simulink model "AM_07_model_pretvornik_FOC"  (R2016a)
settings: Solver=ode23  StartTime=0.0  StopTime=1  FixedStep=25e-9  MaxStep=1/(20*Fstikalna)  RelTol=1e-2
InitFcn:
  | parametriAM
values from neighbouring files (symbols this model uses):
  Imrn = 7.4    [parametriAM.m]
  In = 12.7    [parametriAM.m]
  Ismax = In*sqrt(2)    [parametriAM.m]
  J = 0.019    [parametriAM.m]    (also in podatki.m = 0.01)
  Ki_tok = 5.0    (= 5)    [parametriAM.m]
  Ki_wr = 1000    [parametriAM.m]
  Kp_tok = 0.05    [parametriAM.m]
  Kp_wr = 50    [parametriAM.m]
  Lm = 0.0493    [parametriAM.m]    (also in podatki.m = 0.2342)
  Lr = 0.05315    [parametriAM.m]    (also in podatki.m = 0.2449)
  Ls = 0.05315    [parametriAM.m]    (also in podatki.m = 0.2449)
  Lst = sigma*Ls    (= 0.00742111947319)    [parametriAM.m]
  pp = 3    [parametriAM.m]    (also in podatki.m = 2)
  sigma = 1 - 1/((1+sigmaR)*(1+sigmaS))    (= 0.13962595434)    [parametriAM.m]
  Tr = Lr/Rr    (= 0.0771407837446)    [parametriAM.m]
  Tstikalna = 1/Fstikalna    (= 0.0001)    [parametriAM.m]
  Udc = Un*sqrt(2/3*2)    [parametriAM.m]
  Un = 216    [parametriAM.m]
  wb_upper_limit_field_weaking = sqrt((Ls^2+Lst^2)/(2*Lst^2*Ls^2))*Un/Ismax    [parametriAM.m]
  wn = Udc/sqrt(Ls^2*(Imrn)^2+Lst^2*(Ismax^2-(Imrn)^2))    [maximalnaelipsa.m]    (also in parametriAM.m = Udc/sqrt(Ls^2*(Imrn)^2+Lst^2*(Ismax^2-(Imrn)^2))/pp/sqrt(2))
undefined symbols (not defined in the file or in its folder): DiscIntNeverNeededParam
undefined symbols (not defined in the file): Rr, Rs
libraries: simulink x23, simulink_extras x3
(part 1 of 2)
settings Model: Creator=Mitja  LastModifiedBy=Mitja1
settings DataIOCC: LimitDataPoints=on  SaveFormat=Array  SignalLoggingSaveFormat=ModelDataLogs
settings OptimizationCC: ExpressionDepthLimit=2147483647  InitFltsAndDblsToZero=on
settings DebuggingCC: SaveWithParameterizedLinksMsg=none  UnderspecifiedInitializationDetection=Classic  MergeDetectMultiDrivingBlocksExec=none  SignalResolutionControl=TryResolveAllWithWarning  SolverPrmCheckMsg=warning  FcnCallInpInsideContextMsg=UseLocalSettings  StateNameClashWarn=warning  StrictBusMsg=Warning
settings HardwareCC: ProdBitPerPointer=32  ProdLargestAtomicFloat=None  ProdIntDivRoundTo=Undefined  ProdEndianess=Unspecified  ProdWordSize=32  ProdHWDeviceType=32-bit Generic
settings ModelReferenceCC: PropagateSignalLabelsOutOfModel=off
settings GRTTargetCC: TargetFcnLib=ansi_tfl_tmw.mat  CombineOutputUpdateFcns=off  GRTInterface=on
settings ConfigComp: CovModelRefEnable=Off

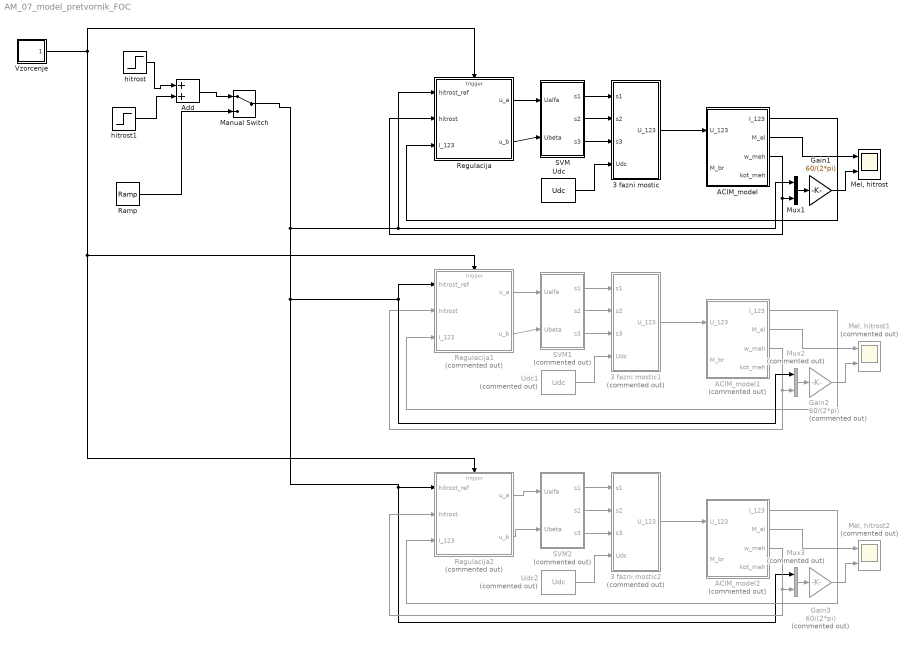
== system AM_07_model_pretvornik_FOC ==
  3 fazni mostic : Subsystem
  3 fazni mostic1 : Subsystem  Commented=on
  3 fazni mostic2 : Subsystem  Commented=on
  ACIM_model : Subsystem  mask{R_s=Rs, R_r=Rr, L_s=Ls, L_r=Lr, L_m=Lm, sigma=sigma, pp=pp, J=J, Ktrenja=0, Kupora=0}
      mask prompts: R_s "Statorska upornost"; R_r "Rotorska upornost"; L_s "Statorska induktivnost"; L_r "Rotorska induktivnost"; L_m "Medsebojna induktivnost"; sigma "Fakstor stresanja"; pp "Število polovih parov"; J "Mehanska vztrajnost"; Ktrenja "Koeficient trenja"; Kupora "Koeficient upora"
  ACIM_model1 : Subsystem  Commented=on  mask{R_s=Rs, R_r=Rr, L_s=Ls, L_r=Lr, L_m=Lm, sigma=sigma, pp=pp, J=J, Ktrenja=0, Kupora=0}
      mask prompts: R_s "Statorska upornost"; R_r "Rotorska upornost"; L_s "Statorska induktivnost"; L_r "Rotorska induktivnost"; L_m "Medsebojna induktivnost"; sigma "Fakstor stresanja"; pp "Število polovih parov"; J "Mehanska vztrajnost"; Ktrenja "Koeficient trenja"; Kupora "Koeficient upora"
  ACIM_model2 : Subsystem  Commented=on  mask{R_s=Rs, R_r=Rr, L_s=Ls, L_r=Lr, L_m=Lm, sigma=sigma, pp=pp, J=J, Ktrenja=0, Kupora=0}
      mask prompts: R_s "Statorska upornost"; R_r "Rotorska upornost"; L_s "Statorska induktivnost"; L_r "Rotorska induktivnost"; L_m "Medsebojna induktivnost"; sigma "Fakstor stresanja"; pp "Število polovih parov"; J "Mehanska vztrajnost"; Ktrenja "Koeficient trenja"; Kupora "Koeficient upora"
  Add : Sum
  Gain1 : Gain  Gain=60/(2*pi)
  Gain2 : Gain  Commented=on  Gain=60/(2*pi)
  Gain3 : Gain  Commented=on  Gain=60/(2*pi)
  Manual Switch : ManualSwitch
  "Mel, hitrost" : Scope  NumInputPorts=2
  "Mel, hitrost1" : Scope  Commented=on  NumInputPorts=2
  "Mel, hitrost2" : Scope  Commented=on  NumInputPorts=2
  Mux1 : Mux  Inputs=2
  Mux2 : Mux  Commented=on  Inputs=2
  Mux3 : Mux  Commented=on  Inputs=2
  Ramp : simulink/Sources/Ramp  slope=1  start=0  X0=0
  Regulacija : Subsystem  TreatAsAtomicUnit=on
  Regulacija1 : Subsystem  Commented=on  TreatAsAtomicUnit=on
  Regulacija2 : Subsystem  Commented=on  TreatAsAtomicUnit=on
  SVM : Subsystem
  SVM1 : Subsystem  Commented=on
  SVM2 : Subsystem  Commented=on
  Udc : Constant  Value=Udc
  Udc1 : Constant  Commented=on  Value=Udc
  Udc2 : Constant  Commented=on  Value=Udc
  Vzorcenje : Subsystem
  hitrost : Step  Time=0.1  After=(2000)*2*pi/60  SampleTime=0
  hitrost1 : Step  Time=0.3  After=2000*2*pi/60  SampleTime=0
  wires:
  Udc/1 -> 3 fazni mostic/4(Udc)
  SVM/1(s1) -> 3 fazni mostic/1(s1)
  SVM/2(s2) -> 3 fazni mostic/2(s2)
  SVM/3(s3) -> 3 fazni mostic/3(s3)
  Regulacija/1(u_a) -> SVM/1(Ualfa)
  Regulacija/2(u_b) -> SVM/2(Ubeta)
  3 fazni mostic/1(U_123) -> ACIM_model/1(U_123)
  hitrost/1 -> Add/1
  ACIM_model/1(I_123) -> Regulacija/3(I_123)
  ACIM_model/2(M_el) -> "Mel, hitrost"/1
  ACIM_model/3(w_meh) -> Mux1/2, Regulacija/2(hitrost)
  Gain1/1 -> "Mel, hitrost"/2
  Mux1/1 -> Gain1/1
  Udc1/1 -> 3 fazni mostic1/4(Udc)
  SVM1/1(s1) -> 3 fazni mostic1/1(s1)
  SVM1/2(s2) -> 3 fazni mostic1/2(s2)
  SVM1/3(s3) -> 3 fazni mostic1/3(s3)
  Regulacija1/1(u_a) -> SVM1/1(Ualfa)
  Regulacija1/2(u_b) -> SVM1/2(Ubeta)
  3 fazni mostic1/1(U_123) -> ACIM_model1/1(U_123)
  ACIM_model1/1(I_123) -> Regulacija1/3(I_123)
  ACIM_model1/2(M_el) -> "Mel, hitrost1"/1
  ACIM_model1/3(w_meh) -> Regulacija1/2(hitrost), Mux2/2
  Gain2/1 -> "Mel, hitrost1"/2
  Mux2/1 -> Gain2/1
  Udc2/1 -> 3 fazni mostic2/4(Udc)
  SVM2/1(s1) -> 3 fazni mostic2/1(s1)
  SVM2/2(s2) -> 3 fazni mostic2/2(s2)
  SVM2/3(s3) -> 3 fazni mostic2/3(s3)
  Regulacija2/1(u_a) -> SVM2/1(Ualfa)
  Regulacija2/2(u_b) -> SVM2/2(Ubeta)
  3 fazni mostic2/1(U_123) -> ACIM_model2/1(U_123)
  Manual Switch/1 -> Mux3/1, Regulacija2/1(hitrost_ref), Mux2/1, Regulacija1/1(hitrost_ref), Regulacija/1(hitrost_ref), Mux1/1
  ACIM_model2/1(I_123) -> Regulacija2/3(I_123)
  ACIM_model2/2(M_el) -> "Mel, hitrost2"/1
  ACIM_model2/3(w_meh) -> Mux3/2, Regulacija2/2(hitrost)
  Vzorcenje/1(trigger) -> Regulacija/Trigger, Regulacija2/Trigger, Regulacija1/Trigger
  Gain3/1 -> "Mel, hitrost2"/2
  Mux3/1 -> Gain3/1
  Ramp/1 -> Manual Switch/2
  Add/1 -> Manual Switch/1
  hitrost1/1 -> Add/2

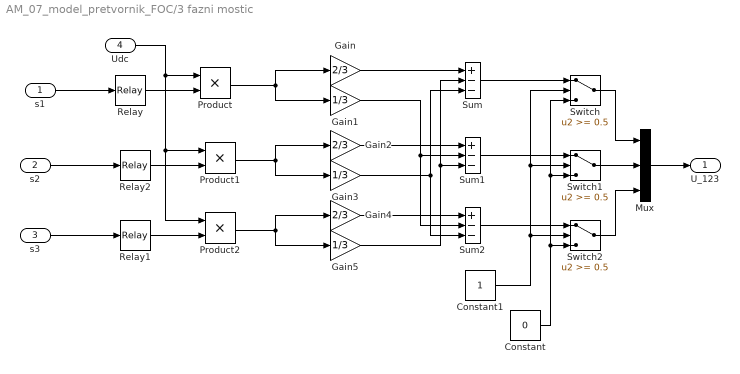
== system AM_07_model_pretvornik_FOC/3 fazni mostic ==
  s1 : Inport
  s2 : Inport  Port=2
  s3 : Inport  Port=3
  Udc : Inport  Port=4
  Constant : Constant  Value=0
  Constant1 : Constant
  Gain : Gain  Gain=2/3
  Gain1 : Gain  Gain=1/3
  Gain2 : Gain  Gain=2/3
  Gain3 : Gain  Gain=1/3
  Gain4 : Gain  Gain=2/3
  Gain5 : Gain  Gain=1/3
  Mux : Mux  Inputs=3
  Product : Product  RndMeth=Zero
  Product1 : Product  RndMeth=Zero
  Product2 : Product  RndMeth=Zero
  Relay : Relay  OnSwitchValue=0.5  OffSwitchValue=0.5  OnOutputValue=0.5  OffOutputValue=-0.5
  Relay1 : Relay  OnSwitchValue=0.5  OffSwitchValue=0.5  OnOutputValue=0.5  OffOutputValue=-0.5
  Relay2 : Relay  OnSwitchValue=0.5  OffSwitchValue=0.5  OnOutputValue=0.5  OffOutputValue=-0.5
  Sum : Sum  Inputs=+--
  Sum1 : Sum  Inputs=+--
  Sum2 : Sum  Inputs=+--
  Switch : Switch  Threshold=0.5
  Switch1 : Switch  Threshold=0.5
  Switch2 : Switch  Threshold=0.5
  U_123 : Outport
  wires:
  Constant/1 -> Switch2/3, Switch1/3, Switch/3
  Constant1/1 -> Switch2/2, Switch1/2, Switch/2
  Udc/1 -> Product/1, Product1/1, Product2/1
  Sum/1 -> Switch/1
  Sum1/1 -> Switch1/1
  Sum2/1 -> Switch2/1
  Product/1 -> Gain/1, Gain1/1
  Product1/1 -> Gain2/1, Gain3/1
  Product2/1 -> Gain4/1, Gain5/1
  Gain/1 -> Sum/1
  Gain2/1 -> Sum1/1
  Gain4/1 -> Sum2/1
  Gain1/1 -> Sum2/2, Sum1/2
  Gain3/1 -> Sum2/3, Sum/3
  Gain5/1 -> Sum/2, Sum1/3
  Relay/1 -> Product/2
  Relay2/1 -> Product1/2
  Relay1/1 -> Product2/2
  s3/1 -> Relay1/1
  s1/1 -> Relay/1
  s2/1 -> Relay2/1
  Switch1/1 -> Mux/2
  Switch/1 -> Mux/1
  Switch2/1 -> Mux/3
  Mux/1 -> U_123/1

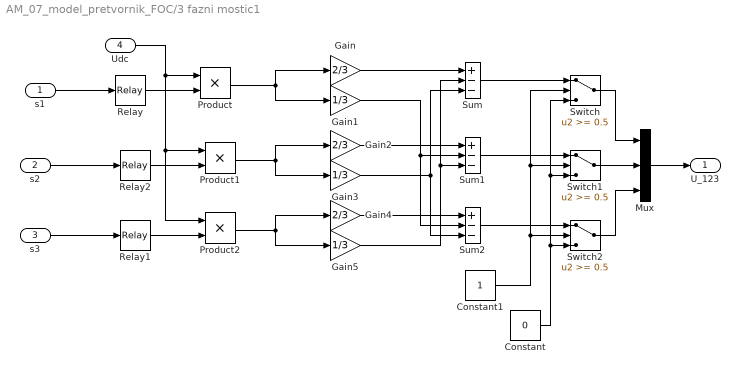
== system AM_07_model_pretvornik_FOC/3 fazni mostic1 ==
  s1 : Inport
  s2 : Inport  Port=2
  s3 : Inport  Port=3
  Udc : Inport  Port=4
  Constant : Constant  Value=0
  Constant1 : Constant
  Gain : Gain  Gain=2/3
  Gain1 : Gain  Gain=1/3
  Gain2 : Gain  Gain=2/3
  Gain3 : Gain  Gain=1/3
  Gain4 : Gain  Gain=2/3
  Gain5 : Gain  Gain=1/3
  Mux : Mux  Inputs=3
  Product : Product  RndMeth=Zero
  Product1 : Product  RndMeth=Zero
  Product2 : Product  RndMeth=Zero
  Relay : Relay  OnSwitchValue=0.5  OffSwitchValue=0.5  OnOutputValue=0.5  OffOutputValue=-0.5
  Relay1 : Relay  OnSwitchValue=0.5  OffSwitchValue=0.5  OnOutputValue=0.5  OffOutputValue=-0.5
  Relay2 : Relay  OnSwitchValue=0.5  OffSwitchValue=0.5  OnOutputValue=0.5  OffOutputValue=-0.5
  Sum : Sum  Inputs=+--
  Sum1 : Sum  Inputs=+--
  Sum2 : Sum  Inputs=+--
  Switch : Switch  Threshold=0.5
  Switch1 : Switch  Threshold=0.5
  Switch2 : Switch  Threshold=0.5
  U_123 : Outport
  wires:
  Mux/1 -> U_123/1
  Switch2/1 -> Mux/3
  Switch/1 -> Mux/1
  Switch1/1 -> Mux/2
  s2/1 -> Relay2/1
  s1/1 -> Relay/1
  s3/1 -> Relay1/1
  Relay1/1 -> Product2/2
  Relay2/1 -> Product1/2
  Relay/1 -> Product/2
  Gain5/1 -> Sum1/3, Sum/2
  Gain3/1 -> Sum/3, Sum2/3
  Gain1/1 -> Sum1/2, Sum2/2
  Gain4/1 -> Sum2/1
  Gain2/1 -> Sum1/1
  Gain/1 -> Sum/1
  Product2/1 -> Gain5/1, Gain4/1
  Product1/1 -> Gain3/1, Gain2/1
  Product/1 -> Gain1/1, Gain/1
  Sum2/1 -> Switch2/1
  Sum1/1 -> Switch1/1
  Sum/1 -> Switch/1
  Udc/1 -> Product2/1, Product1/1, Product/1
  Constant1/1 -> Switch/2, Switch1/2, Switch2/2
  Constant/1 -> Switch/3, Switch1/3, Switch2/3

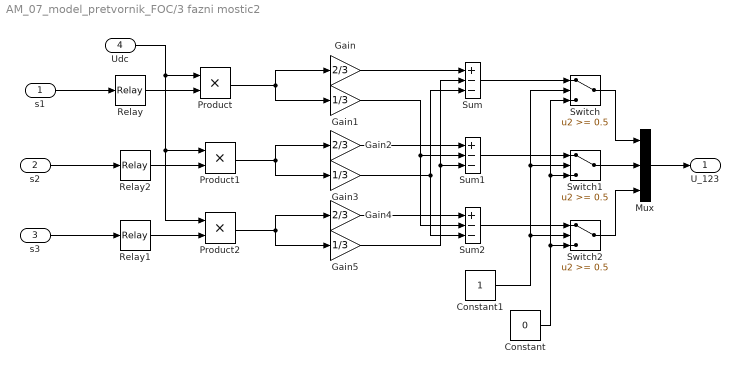
== system AM_07_model_pretvornik_FOC/3 fazni mostic2 ==
  s1 : Inport
  s2 : Inport  Port=2
  s3 : Inport  Port=3
  Udc : Inport  Port=4
  Constant : Constant  Value=0
  Constant1 : Constant
  Gain : Gain  Gain=2/3
  Gain1 : Gain  Gain=1/3
  Gain2 : Gain  Gain=2/3
  Gain3 : Gain  Gain=1/3
  Gain4 : Gain  Gain=2/3
  Gain5 : Gain  Gain=1/3
  Mux : Mux  Inputs=3
  Product : Product  RndMeth=Zero
  Product1 : Product  RndMeth=Zero
  Product2 : Product  RndMeth=Zero
  Relay : Relay  OnSwitchValue=0.5  OffSwitchValue=0.5  OnOutputValue=0.5  OffOutputValue=-0.5
  Relay1 : Relay  OnSwitchValue=0.5  OffSwitchValue=0.5  OnOutputValue=0.5  OffOutputValue=-0.5
  Relay2 : Relay  OnSwitchValue=0.5  OffSwitchValue=0.5  OnOutputValue=0.5  OffOutputValue=-0.5
  Sum : Sum  Inputs=+--
  Sum1 : Sum  Inputs=+--
  Sum2 : Sum  Inputs=+--
  Switch : Switch  Threshold=0.5
  Switch1 : Switch  Threshold=0.5
  Switch2 : Switch  Threshold=0.5
  U_123 : Outport
  wires:
  Constant/1 -> Switch2/3, Switch1/3, Switch/3
  Constant1/1 -> Switch2/2, Switch1/2, Switch/2
  Udc/1 -> Product/1, Product1/1, Product2/1
  Sum/1 -> Switch/1
  Sum1/1 -> Switch1/1
  Sum2/1 -> Switch2/1
  Product/1 -> Gain/1, Gain1/1
  Product1/1 -> Gain2/1, Gain3/1
  Product2/1 -> Gain4/1, Gain5/1
  Gain/1 -> Sum/1
  Gain2/1 -> Sum1/1
  Gain4/1 -> Sum2/1
  Gain1/1 -> Sum2/2, Sum1/2
  Gain3/1 -> Sum2/3, Sum/3
  Gain5/1 -> Sum/2, Sum1/3
  Relay/1 -> Product/2
  Relay2/1 -> Product1/2
  Relay1/1 -> Product2/2
  s3/1 -> Relay1/1
  s1/1 -> Relay/1
  s2/1 -> Relay2/1
  Switch1/1 -> Mux/2
  Switch/1 -> Mux/1
  Switch2/1 -> Mux/3
  Mux/1 -> U_123/1

== system AM_07_model_pretvornik_FOC/ACIM_model ==
  U_123 : Inport
  M_br : Inport  Port=2
  Elektricni del1 : Subsystem  mask{Rs=R_s, Rr=R_r, Ls=L_s, Lr=L_r, Lm=L_m, sigma=sigma, pp=pp}
      mask prompts: Rs "Statorska upornost"; Rr "Rotorska upornost"; Ls "Statorska induktivnost"; Lr "Statorska induktivnost"; Lm "Medsebojna induktivnost"; sigma "Faktor stresanja sigma"; pp "Število polovih parov"
  Mehanika : Subsystem  mask{J=J, Ktrenja=Ktrenja, Kupora=Kupora}
      mask prompts: J "Rotacijska vztrajnost"; Ktrenja "Koeficient trenja"; Kupora "Koeficient zracnega upora"
  I_123 : Outport
  M_el : Outport  Port=2
  w_meh : Outport  Port=3
  kot_meh : Outport  Port=4
  wires:
  Mehanika/1(w_meh) -> Elektricni del1/2(w_meh), w_meh/1
  Mehanika/2(kot_meh) -> kot_meh/1
  Elektricni del1/2(I_123) -> I_123/1
  U_123/1 -> Elektricni del1/1(U_123)
  M_br/1 -> Mehanika/2(M_br)
  Elektricni del1/1(Mel) -> M_el/1, Mehanika/1(M_el)

== system AM_07_model_pretvornik_FOC/ACIM_model1 ==
  U_123 : Inport
  M_br : Inport  Port=2
  Elektricni del1 : Subsystem  mask{Rs=R_s, Rr=R_r, Ls=L_s, Lr=L_r, Lm=L_m, sigma=sigma, pp=pp}
      mask prompts: Rs "Statorska upornost"; Rr "Rotorska upornost"; Ls "Statorska induktivnost"; Lr "Statorska induktivnost"; Lm "Medsebojna induktivnost"; sigma "Faktor stresanja sigma"; pp "Število polovih parov"
  Mehanika : Subsystem  mask{J=J, Ktrenja=Ktrenja, Kupora=Kupora}
      mask prompts: J "Rotacijska vztrajnost"; Ktrenja "Koeficient trenja"; Kupora "Koeficient zracnega upora"
  I_123 : Outport
  M_el : Outport  Port=2
  w_meh : Outport  Port=3
  kot_meh : Outport  Port=4
  wires:
  Elektricni del1/1(Mel) -> Mehanika/1(M_el), M_el/1
  M_br/1 -> Mehanika/2(M_br)
  U_123/1 -> Elektricni del1/1(U_123)
  Elektricni del1/2(I_123) -> I_123/1
  Mehanika/2(kot_meh) -> kot_meh/1
  Mehanika/1(w_meh) -> w_meh/1, Elektricni del1/2(w_meh)

== system AM_07_model_pretvornik_FOC/ACIM_model2 ==
  U_123 : Inport
  M_br : Inport  Port=2
  Elektricni del1 : Subsystem  mask{Rs=R_s, Rr=R_r, Ls=L_s, Lr=L_r, Lm=L_m, sigma=sigma, pp=pp}
      mask prompts: Rs "Statorska upornost"; Rr "Rotorska upornost"; Ls "Statorska induktivnost"; Lr "Statorska induktivnost"; Lm "Medsebojna induktivnost"; sigma "Faktor stresanja sigma"; pp "Število polovih parov"
  Mehanika : Subsystem  mask{J=J, Ktrenja=Ktrenja, Kupora=Kupora}
      mask prompts: J "Rotacijska vztrajnost"; Ktrenja "Koeficient trenja"; Kupora "Koeficient zracnega upora"
  I_123 : Outport
  M_el : Outport  Port=2
  w_meh : Outport  Port=3
  kot_meh : Outport  Port=4
  wires:
  Mehanika/1(w_meh) -> Elektricni del1/2(w_meh), w_meh/1
  Mehanika/2(kot_meh) -> kot_meh/1
  Elektricni del1/2(I_123) -> I_123/1
  U_123/1 -> Elektricni del1/1(U_123)
  M_br/1 -> Mehanika/2(M_br)
  Elektricni del1/1(Mel) -> M_el/1, Mehanika/1(M_el)

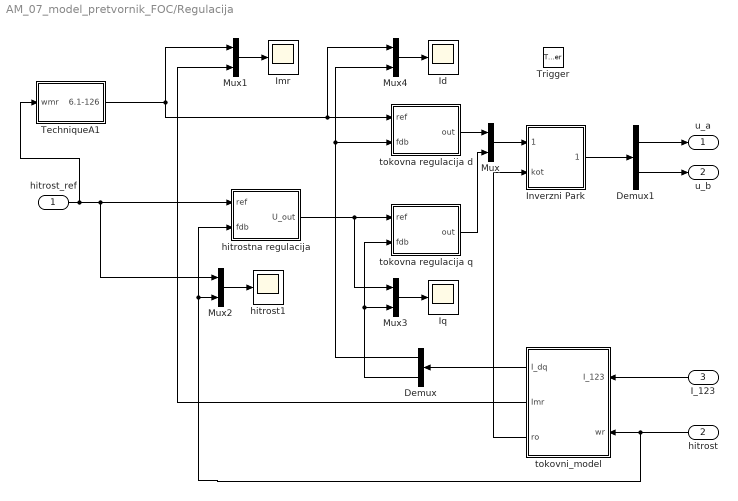
== system AM_07_model_pretvornik_FOC/Regulacija ==
  hitrost_ref : Inport
  hitrost : Inport  Port=2
  I_123 : Inport  Port=3
  Trigger : TriggerPort  TriggerType=falling  VariantControl=Variant
  Demux : Demux  Outputs=2
  Demux1 : Demux  Outputs=2
  Id : Scope
  Imr : Scope
  Inverzni Park : Subsystem
  Iq : Scope
  Mux{,1..4} (5 alike) : Mux  Inputs=2
  TechniqueA1 : Subsystem
  hitrost1 : Scope
  hitrostna regulacija : Subsystem
  tokovna regulacija d : Subsystem
  tokovna regulacija q : Subsystem
  tokovni_model : Subsystem
  u_a : Outport
  u_b : Outport  Port=2
  wires:
  I_123/1 -> tokovni_model/1(I_123)
  hitrost/1 -> Mux2/2, hitrostna regulacija/2(fdb), tokovni_model/2(wr)
  tokovni_model/3(ro) -> Inverzni Park/2(kot)
  hitrost_ref/1 -> TechniqueA1/1(wmr), hitrostna regulacija/1(ref), Mux2/1
  Mux/1 -> Inverzni Park/1(U_dq)
  TechniqueA1/1(6.1-126) -> tokovna regulacija d/1(ref), Mux4/1, Mux1/1
  tokovna regulacija d/1(out) -> Mux/1
  tokovna regulacija q/1(out) -> Mux/2
  Demux/1 -> tokovna regulacija d/2(fdb), Mux4/2
  Demux/2 -> Mux3/2, tokovna regulacija q/2(fdb)
  Inverzni Park/1(U_ab) -> Demux1/1
  Demux1/1 -> u_a/1
  Demux1/2 -> u_b/1
  Mux1/1 -> Imr/1
  Mux2/1 -> hitrost1/1
  Mux3/1 -> Iq/1
  Mux4/1 -> Id/1
  tokovni_model/2(Imr) -> Mux1/2
  tokovni_model/1(I_dq) -> Demux/1
  hitrostna regulacija/1(U_out) -> tokovna regulacija q/1(ref), Mux3/1

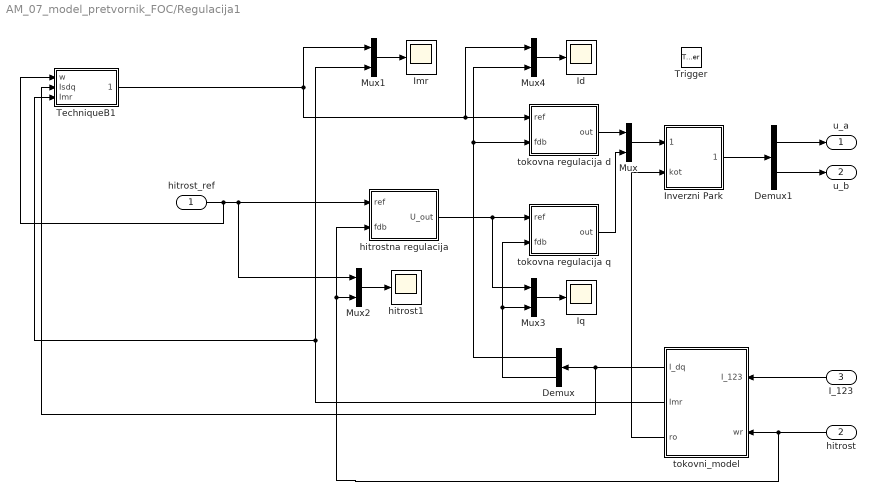
== system AM_07_model_pretvornik_FOC/Regulacija1 ==
  hitrost_ref : Inport
  hitrost : Inport  Port=2
  I_123 : Inport  Port=3
  Trigger : TriggerPort  TriggerType=falling  VariantControl=Variant
  Demux : Demux  Outputs=2
  Demux1 : Demux  Outputs=2
  Id : Scope
  Imr : Scope
  Inverzni Park : Subsystem
  Iq : Scope
  Mux{,1..4} (5 alike) : Mux  Inputs=2
  TechniqueB1 : Subsystem
  hitrost1 : Scope
  hitrostna regulacija : Subsystem
  tokovna regulacija d : Subsystem
  tokovna regulacija q : Subsystem
  tokovni_model : Subsystem
  u_a : Outport
  u_b : Outport  Port=2
  wires:
  hitrostna regulacija/1(U_out) -> Mux3/1, tokovna regulacija q/1(ref)
  tokovni_model/1(I_dq) -> TechniqueB1/2(Isdq), Demux/1
  tokovni_model/2(Imr) -> TechniqueB1/3(Imr), Mux1/2
  Mux4/1 -> Id/1
  Mux3/1 -> Iq/1
  Mux2/1 -> hitrost1/1
  Mux1/1 -> Imr/1
  Demux1/2 -> u_b/1
  Demux1/1 -> u_a/1
  Inverzni Park/1(U_ab) -> Demux1/1
  Demux/2 -> tokovna regulacija q/2(fdb), Mux3/2
  Demux/1 -> Mux4/2, tokovna regulacija d/2(fdb)
  tokovna regulacija q/1(out) -> Mux/2
  tokovna regulacija d/1(out) -> Mux/1
  TechniqueB1/1(6.1-135) -> Mux4/1, tokovna regulacija d/1(ref), Mux1/1
  Mux/1 -> Inverzni Park/1(U_dq)
  hitrost_ref/1 -> TechniqueB1/1(w), Mux2/1, hitrostna regulacija/1(ref)
  tokovni_model/3(ro) -> Inverzni Park/2(kot)
  hitrost/1 -> tokovni_model/2(wr), hitrostna regulacija/2(fdb), Mux2/2
  I_123/1 -> tokovni_model/1(I_123)

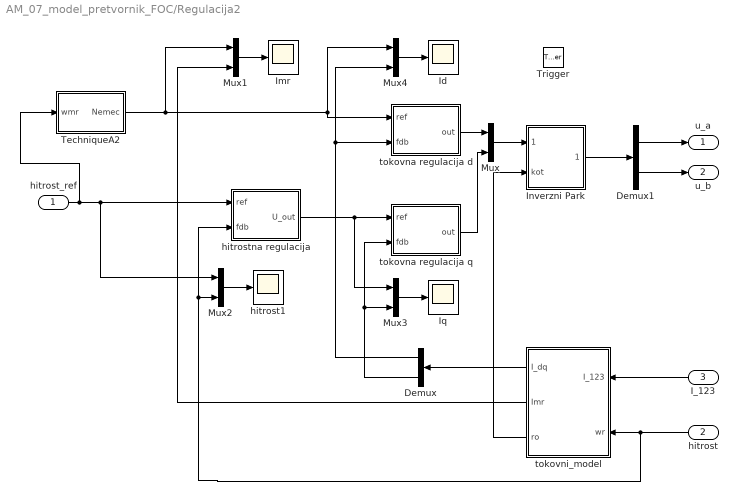
== system AM_07_model_pretvornik_FOC/Regulacija2 ==
  hitrost_ref : Inport
  hitrost : Inport  Port=2
  I_123 : Inport  Port=3
  Trigger : TriggerPort  TriggerType=falling  VariantControl=Variant
  Demux : Demux  Outputs=2
  Demux1 : Demux  Outputs=2
  Id : Scope
  Imr : Scope
  Inverzni Park : Subsystem
  Iq : Scope
  Mux{,1..4} (5 alike) : Mux  Inputs=2
  TechniqueA2 : Subsystem
  hitrost1 : Scope
  hitrostna regulacija : Subsystem
  tokovna regulacija d : Subsystem
  tokovna regulacija q : Subsystem
  tokovni_model : Subsystem
  u_a : Outport
  u_b : Outport  Port=2
  wires:
  I_123/1 -> tokovni_model/1(I_123)
  hitrost/1 -> Mux2/2, hitrostna regulacija/2(fdb), tokovni_model/2(wr)
  tokovni_model/3(ro) -> Inverzni Park/2(kot)
  hitrost_ref/1 -> TechniqueA2/1(wmr), hitrostna regulacija/1(ref), Mux2/1
  Mux/1 -> Inverzni Park/1(U_dq)
  TechniqueA2/1(Nemec) -> tokovna regulacija d/1(ref), Mux4/1, Mux1/1
  tokovna regulacija d/1(out) -> Mux/1
  tokovna regulacija q/1(out) -> Mux/2
  Demux/1 -> tokovna regulacija d/2(fdb), Mux4/2
  Demux/2 -> Mux3/2, tokovna regulacija q/2(fdb)
  Inverzni Park/1(U_ab) -> Demux1/1
  Demux1/1 -> u_a/1
  Demux1/2 -> u_b/1
  Mux1/1 -> Imr/1
  Mux2/1 -> hitrost1/1
  Mux3/1 -> Iq/1
  Mux4/1 -> Id/1
  tokovni_model/2(Imr) -> Mux1/2
  tokovni_model/1(I_dq) -> Demux/1
  hitrostna regulacija/1(U_out) -> tokovna regulacija q/1(ref), Mux3/1

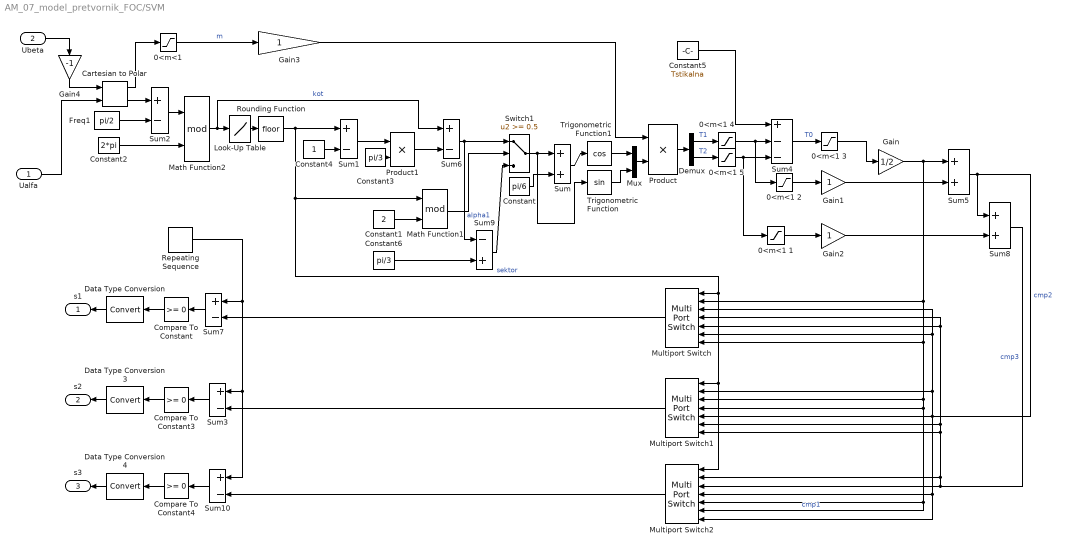
== system AM_07_model_pretvornik_FOC/SVM ==
  Ualfa : Inport
  Ubeta : Inport  Port=2
  "0<m<1 " : Saturate  UpperLimit=0.99  LowerLimit=0
  0<m<1 {1..5} (5 alike) : Saturate  UpperLimit=1  LowerLimit=0
  Cartesian to Polar : simulink_extras/Transformations/Cartesian to Polar
  Compare To Constant : simulink/Logic and Bit Operations/Compare To Constant  relop=>=  const=0  OutDataTypeStr=uint8  ZeroCross=off
  Compare To Constant3 : simulink/Logic and Bit Operations/Compare To Constant  relop=>=  const=0  OutDataTypeStr=uint8  ZeroCross=off
  Compare To Constant4 : simulink/Logic and Bit Operations/Compare To Constant  relop=>=  const=0  OutDataTypeStr=uint8  ZeroCross=off
  Constant : Constant  Value=pi/6
  Constant1 : Constant  Value=2
  Constant2 : Constant  Value=2*pi
  Constant3 : Constant  Value=pi/3
  Constant4 : Constant
  Constant5 : Constant  Value=Tstikalna
  Constant6 : Constant  Value=pi/3
  Data Type Conversion : DataTypeConversion
  Data Type Conversion3 : DataTypeConversion
  Data Type Conversion4 : DataTypeConversion
  Demux : Demux  Outputs=2
  Freq1 : Constant  Value=pi/2
  Gain : Gain  Gain=1/2
  Gain1 : Gain
  Gain2 : Gain
  Gain3 : Gain
  Gain4 : Gain  Gain=-1
  Look-Up Table : Lookup  InputValues=[0:pi/3:5*pi/3]  Table=[1:6]  SaturateOnIntegerOverflow=on
  Math Function1 : Math  Operator=mod  SaturateOnIntegerOverflow=on
  Math Function2 : Math  Operator=mod  SaturateOnIntegerOverflow=on
  Multiport Switch : MultiPortSwitch  Inputs=6  DiagnosticForDefault=Warning
  Multiport Switch1 : MultiPortSwitch  Inputs=6  DiagnosticForDefault=Warning
  Multiport Switch2 : MultiPortSwitch  Inputs=6  DiagnosticForDefault=Warning
  Mux : Mux  Inputs=2
  Product : Product  SaturateOnIntegerOverflow=on  OutDataTypeStr=Inherit: Same as first input
  Product1 : Product  SaturateOnIntegerOverflow=on  OutDataTypeStr=Inherit: Same as first input
  Repeating Sequence : simulink/Sources/Repeating Sequence  rep_seq_t=[0 Tstikalna/2 Tstikalna]  rep_seq_y=[0 1 0]
  Rounding Function : Rounding
  Sum : Sum  SaturateOnIntegerOverflow=on
  Sum1 : Sum  Inputs=+-  SaturateOnIntegerOverflow=on
  Sum10 : Sum  Inputs=+-
  Sum2 : Sum  Inputs=+-  SaturateOnIntegerOverflow=on  InputSameDT=on  OutDataTypeStr=Inherit: Same as first input
  Sum3 : Sum  Inputs=+-
  Sum4 : Sum  Inputs=+--  SaturateOnIntegerOverflow=on
  Sum5 : Sum  SaturateOnIntegerOverflow=on
  Sum6 : Sum  Inputs=+-  SaturateOnIntegerOverflow=on
  Sum7 : Sum  Inputs=+-
  Sum8 : Sum  SaturateOnIntegerOverflow=on
  Sum9 : Sum  Inputs=-+  SaturateOnIntegerOverflow=on
  Switch1 : Switch  Threshold=0.5  SaturateOnIntegerOverflow=on
  Trigonometric Function : Trigonometry
  Trigonometric Function1 : Trigonometry  Operator=cos
  s1 : Outport
  s2 : Outport  Port=2
  s3 : Outport  Port=3
  wires:
  Sum7/1 -> Compare To Constant/1
  Compare To Constant/1 -> Data Type Conversion/1
  Data Type Conversion/1 -> s1/1
  Sum3/1 -> Compare To Constant3/1
  Compare To Constant3/1 -> Data Type Conversion3/1
  Data Type Conversion3/1 -> s2/1
  Sum10/1 -> Compare To Constant4/1
  Compare To Constant4/1 -> Data Type Conversion4/1
  Data Type Conversion4/1 -> s3/1
  Repeating Sequence/1 -> Sum7/1, Sum3/1, Sum10/1
  Cartesian to Polar/1 -> "0<m<1 "/1
  Constant2/1 -> Math Function2/2
  Cartesian to Polar/2 -> Sum2/1
  Freq1/1 -> Sum2/2
  Sum2/1 -> Math Function2/1
  "0<m<1 "/1 -> Gain3/1  "m"
  Math Function2/1 -> Look-Up Table/1, Sum6/1  "kot"
  Look-Up Table/1 -> Rounding Function/1
  Rounding Function/1 -> Sum1/1, Multiport Switch1/1, Multiport Switch2/1, Multiport Switch/1, Math Function1/1  "sektor"
  Trigonometric Function1/1 -> Mux/1
  Trigonometric Function/1 -> Mux/2
  Mux/1 -> Product/2
  Sum/1 -> Trigonometric Function1/1
  Sum1/1 -> Product1/1
  Constant3/1 -> Product1/2
  Constant4/1 -> Sum1/2
  Product1/1 -> Sum6/2
  Constant/1 -> Sum/2
  Multiport Switch/1 -> Sum7/2
  Multiport Switch1/1 -> Sum3/2
  Multiport Switch2/1 -> Sum10/2
  Product/1 -> Demux/1
  Demux/1 -> 0<m<1 4/1  "T1"
  Demux/2 -> 0<m<1 5/1  "T2"
  Constant5/1 -> Sum4/1
  Sum4/1 -> 0<m<1 3/1  "T0"
  Gain1/1 -> Sum5/2
  Gain/1 -> Sum5/1, Multiport Switch/2, Multiport Switch/7, Multiport Switch1/3, Multiport Switch1/4, Multiport Switch2/5, Multiport Switch2/6  "cmp1"
  Sum5/1 -> Sum8/1, Multiport Switch1/5, Multiport Switch2/4, Multiport Switch2/7, Multiport Switch1/2, Multiport Switch/3, Multiport Switch/6  "cmp2"
  Gain2/1 -> Sum8/2
  Sum8/1 -> Multiport Switch/4, Multiport Switch/5, Multiport Switch1/6, Multiport Switch1/7, Multiport Switch2/2, Multiport Switch2/3  "cmp3"
  0<m<1 1/1 -> Gain2/1
  0<m<1 2/1 -> Gain1/1
  0<m<1 3/1 -> Gain/1
  Ubeta/1 -> Gain4/1
  Ualfa/1 -> Cartesian to Polar/2
  Gain3/1 -> Product/1
  Gain4/1 -> Cartesian to Polar/1
  Constant1/1 -> Math Function1/2
  Math Function1/1 -> Switch1/2
  Constant6/1 -> Sum9/2
  Sum9/1 -> Switch1/3
  Switch1/1 -> Trigonometric Function/1, Sum/1
  Sum6/1 -> Switch1/1, Sum9/1  "alpha1"
  0<m<1 4/1 -> Sum4/2, 0<m<1 2/1
  0<m<1 5/1 -> Sum4/3, 0<m<1 1/1

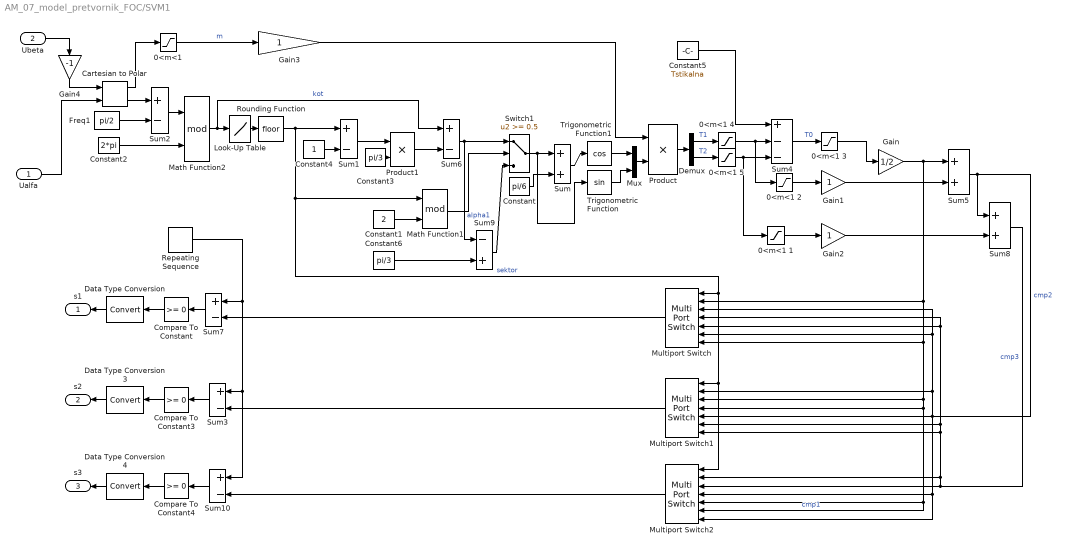
== system AM_07_model_pretvornik_FOC/SVM1 ==
  Ualfa : Inport
  Ubeta : Inport  Port=2
  "0<m<1 " : Saturate  UpperLimit=0.99  LowerLimit=0
  0<m<1 {1..5} (5 alike) : Saturate  UpperLimit=1  LowerLimit=0
  Cartesian to Polar : simulink_extras/Transformations/Cartesian to Polar
  Compare To Constant : simulink/Logic and Bit Operations/Compare To Constant  relop=>=  const=0  OutDataTypeStr=uint8  ZeroCross=off
  Compare To Constant3 : simulink/Logic and Bit Operations/Compare To Constant  relop=>=  const=0  OutDataTypeStr=uint8  ZeroCross=off
  Compare To Constant4 : simulink/Logic and Bit Operations/Compare To Constant  relop=>=  const=0  OutDataTypeStr=uint8  ZeroCross=off
  Constant : Constant  Value=pi/6
  Constant1 : Constant  Value=2
  Constant2 : Constant  Value=2*pi
  Constant3 : Constant  Value=pi/3
  Constant4 : Constant
  Constant5 : Constant  Value=Tstikalna
  Constant6 : Constant  Value=pi/3
  Data Type Conversion : DataTypeConversion
  Data Type Conversion3 : DataTypeConversion
  Data Type Conversion4 : DataTypeConversion
  Demux : Demux  Outputs=2
  Freq1 : Constant  Value=pi/2
  Gain : Gain  Gain=1/2
  Gain1 : Gain
  Gain2 : Gain
  Gain3 : Gain
  Gain4 : Gain  Gain=-1
  Look-Up Table : Lookup  InputValues=[0:pi/3:5*pi/3]  Table=[1:6]  SaturateOnIntegerOverflow=on
  Math Function1 : Math  Operator=mod  SaturateOnIntegerOverflow=on
  Math Function2 : Math  Operator=mod  SaturateOnIntegerOverflow=on
  Multiport Switch : MultiPortSwitch  Inputs=6  DiagnosticForDefault=Warning
  Multiport Switch1 : MultiPortSwitch  Inputs=6  DiagnosticForDefault=Warning
  Multiport Switch2 : MultiPortSwitch  Inputs=6  DiagnosticForDefault=Warning
  Mux : Mux  Inputs=2
  Product : Product  SaturateOnIntegerOverflow=on  OutDataTypeStr=Inherit: Same as first input
  Product1 : Product  SaturateOnIntegerOverflow=on  OutDataTypeStr=Inherit: Same as first input
  Repeating Sequence : simulink/Sources/Repeating Sequence  rep_seq_t=[0 Tstikalna/2 Tstikalna]  rep_seq_y=[0 1 0]
  Rounding Function : Rounding
  Sum : Sum  SaturateOnIntegerOverflow=on
  Sum1 : Sum  Inputs=+-  SaturateOnIntegerOverflow=on
  Sum10 : Sum  Inputs=+-
  Sum2 : Sum  Inputs=+-  SaturateOnIntegerOverflow=on  InputSameDT=on  OutDataTypeStr=Inherit: Same as first input
  Sum3 : Sum  Inputs=+-
  Sum4 : Sum  Inputs=+--  SaturateOnIntegerOverflow=on
  Sum5 : Sum  SaturateOnIntegerOverflow=on
  Sum6 : Sum  Inputs=+-  SaturateOnIntegerOverflow=on
  Sum7 : Sum  Inputs=+-
  Sum8 : Sum  SaturateOnIntegerOverflow=on
  Sum9 : Sum  Inputs=-+  SaturateOnIntegerOverflow=on
  Switch1 : Switch  Threshold=0.5  SaturateOnIntegerOverflow=on
  Trigonometric Function : Trigonometry
  Trigonometric Function1 : Trigonometry  Operator=cos
  s1 : Outport
  s2 : Outport  Port=2
  s3 : Outport  Port=3
  wires:
  0<m<1 5/1 -> 0<m<1 1/1, Sum4/3
  0<m<1 4/1 -> 0<m<1 2/1, Sum4/2
  Sum6/1 -> Sum9/1, Switch1/1  "alpha1"
  Switch1/1 -> Sum/1, Trigonometric Function/1
  Sum9/1 -> Switch1/3
  Constant6/1 -> Sum9/2
  Math Function1/1 -> Switch1/2
  Constant1/1 -> Math Function1/2
  Gain4/1 -> Cartesian to Polar/1
  Gain3/1 -> Product/1
  Ualfa/1 -> Cartesian to Polar/2
  Ubeta/1 -> Gain4/1
  0<m<1 3/1 -> Gain/1
  0<m<1 2/1 -> Gain1/1
  0<m<1 1/1 -> Gain2/1
  Sum8/1 -> Multiport Switch2/3, Multiport Switch2/2, Multiport Switch1/7, Multiport Switch1/6, Multiport Switch/5, Multiport Switch/4  "cmp3"
  Gain2/1 -> Sum8/2
  Sum5/1 -> Multiport Switch/6, Multiport Switch/3, Multiport Switch1/2, Multiport Switch2/7, Multiport Switch2/4, Multiport Switch1/5, Sum8/1  "cmp2"
  Gain/1 -> Multiport Switch2/6, Multiport Switch2/5, Multiport Switch1/4, Multiport Switch1/3, Multiport Switch/7, Multiport Switch/2, Sum5/1  "cmp1"
  Gain1/1 -> Sum5/2
  Sum4/1 -> 0<m<1 3/1  "T0"
  Constant5/1 -> Sum4/1
  Demux/2 -> 0<m<1 5/1  "T2"
  Demux/1 -> 0<m<1 4/1  "T1"
  Product/1 -> Demux/1
  Multiport Switch2/1 -> Sum10/2
  Multiport Switch1/1 -> Sum3/2
  Multiport Switch/1 -> Sum7/2
  Constant/1 -> Sum/2
  Product1/1 -> Sum6/2
  Constant4/1 -> Sum1/2
  Constant3/1 -> Product1/2
  Sum1/1 -> Product1/1
  Sum/1 -> Trigonometric Function1/1
  Mux/1 -> Product/2
  Trigonometric Function/1 -> Mux/2
  Trigonometric Function1/1 -> Mux/1
  Rounding Function/1 -> Math Function1/1, Multiport Switch/1, Multiport Switch2/1, Multiport Switch1/1, Sum1/1  "sektor"
  Look-Up Table/1 -> Rounding Function/1
  Math Function2/1 -> Sum6/1, Look-Up Table/1  "kot"
  "0<m<1 "/1 -> Gain3/1  "m"
  Sum2/1 -> Math Function2/1
  Freq1/1 -> Sum2/2
  Cartesian to Polar/2 -> Sum2/1
  Constant2/1 -> Math Function2/2
  Cartesian to Polar/1 -> "0<m<1 "/1
  Repeating Sequence/1 -> Sum10/1, Sum3/1, Sum7/1
  Data Type Conversion4/1 -> s3/1
  Compare To Constant4/1 -> Data Type Conversion4/1
  Sum10/1 -> Compare To Constant4/1
  Data Type Conversion3/1 -> s2/1
  Compare To Constant3/1 -> Data Type Conversion3/1
  Sum3/1 -> Compare To Constant3/1
  Data Type Conversion/1 -> s1/1
  Compare To Constant/1 -> Data Type Conversion/1
  Sum7/1 -> Compare To Constant/1

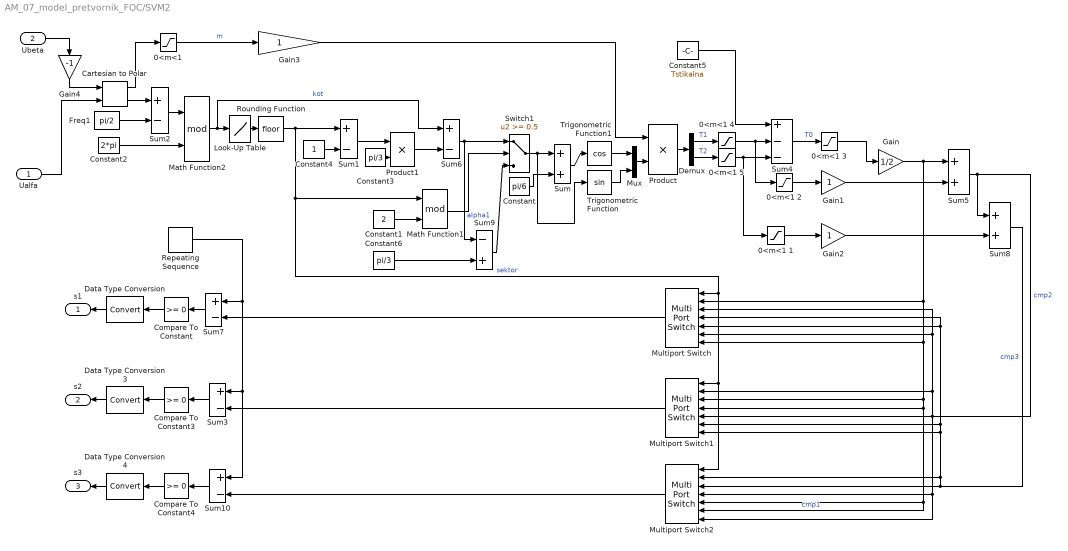
== system AM_07_model_pretvornik_FOC/SVM2 ==
  Ualfa : Inport
  Ubeta : Inport  Port=2
  "0<m<1 " : Saturate  UpperLimit=0.99  LowerLimit=0
  0<m<1 {1..5} (5 alike) : Saturate  UpperLimit=1  LowerLimit=0
  Cartesian to Polar : simulink_extras/Transformations/Cartesian to Polar
  Compare To Constant : simulink/Logic and Bit Operations/Compare To Constant  relop=>=  const=0  OutDataTypeStr=uint8  ZeroCross=off
  Compare To Constant3 : simulink/Logic and Bit Operations/Compare To Constant  relop=>=  const=0  OutDataTypeStr=uint8  ZeroCross=off
  Compare To Constant4 : simulink/Logic and Bit Operations/Compare To Constant  relop=>=  const=0  OutDataTypeStr=uint8  ZeroCross=off
  Constant : Constant  Value=pi/6
  Constant1 : Constant  Value=2
  Constant2 : Constant  Value=2*pi
  Constant3 : Constant  Value=pi/3
  Constant4 : Constant
  Constant5 : Constant  Value=Tstikalna
  Constant6 : Constant  Value=pi/3
  Data Type Conversion : DataTypeConversion
  Data Type Conversion3 : DataTypeConversion
  Data Type Conversion4 : DataTypeConversion
  Demux : Demux  Outputs=2
  Freq1 : Constant  Value=pi/2
  Gain : Gain  Gain=1/2
  Gain1 : Gain
  Gain2 : Gain
  Gain3 : Gain
  Gain4 : Gain  Gain=-1
  Look-Up Table : Lookup  InputValues=[0:pi/3:5*pi/3]  Table=[1:6]  SaturateOnIntegerOverflow=on
  Math Function1 : Math  Operator=mod  SaturateOnIntegerOverflow=on
  Math Function2 : Math  Operator=mod  SaturateOnIntegerOverflow=on
  Multiport Switch : MultiPortSwitch  Inputs=6  DiagnosticForDefault=Warning
  Multiport Switch1 : MultiPortSwitch  Inputs=6  DiagnosticForDefault=Warning
  Multiport Switch2 : MultiPortSwitch  Inputs=6  DiagnosticForDefault=Warning
  Mux : Mux  Inputs=2
  Product : Product  SaturateOnIntegerOverflow=on  OutDataTypeStr=Inherit: Same as first input
  Product1 : Product  SaturateOnIntegerOverflow=on  OutDataTypeStr=Inherit: Same as first input
  Repeating Sequence : simulink/Sources/Repeating Sequence  rep_seq_t=[0 Tstikalna/2 Tstikalna]  rep_seq_y=[0 1 0]
  Rounding Function : Rounding
  Sum : Sum  SaturateOnIntegerOverflow=on
  Sum1 : Sum  Inputs=+-  SaturateOnIntegerOverflow=on
  Sum10 : Sum  Inputs=+-
  Sum2 : Sum  Inputs=+-  SaturateOnIntegerOverflow=on  InputSameDT=on  OutDataTypeStr=Inherit: Same as first input
  Sum3 : Sum  Inputs=+-
  Sum4 : Sum  Inputs=+--  SaturateOnIntegerOverflow=on
  Sum5 : Sum  SaturateOnIntegerOverflow=on
  Sum6 : Sum  Inputs=+-  SaturateOnIntegerOverflow=on
  Sum7 : Sum  Inputs=+-
  Sum8 : Sum  SaturateOnIntegerOverflow=on
  Sum9 : Sum  Inputs=-+  SaturateOnIntegerOverflow=on
  Switch1 : Switch  Threshold=0.5  SaturateOnIntegerOverflow=on
  Trigonometric Function : Trigonometry
  Trigonometric Function1 : Trigonometry  Operator=cos
  s1 : Outport
  s2 : Outport  Port=2
  s3 : Outport  Port=3
  wires:
  Sum7/1 -> Compare To Constant/1
  Compare To Constant/1 -> Data Type Conversion/1
  Data Type Conversion/1 -> s1/1
  Sum3/1 -> Compare To Constant3/1
  Compare To Constant3/1 -> Data Type Conversion3/1
  Data Type Conversion3/1 -> s2/1
  Sum10/1 -> Compare To Constant4/1
  Compare To Constant4/1 -> Data Type Conversion4/1
  Data Type Conversion4/1 -> s3/1
  Repeating Sequence/1 -> Sum7/1, Sum3/1, Sum10/1
  Cartesian to Polar/1 -> "0<m<1 "/1
  Constant2/1 -> Math Function2/2
  Cartesian to Polar/2 -> Sum2/1
  Freq1/1 -> Sum2/2
  Sum2/1 -> Math Function2/1
  "0<m<1 "/1 -> Gain3/1  "m"
  Math Function2/1 -> Look-Up Table/1, Sum6/1  "kot"
  Look-Up Table/1 -> Rounding Function/1
  Rounding Function/1 -> Sum1/1, Multiport Switch1/1, Multiport Switch2/1, Multiport Switch/1, Math Function1/1  "sektor"
  Trigonometric Function1/1 -> Mux/1
  Trigonometric Function/1 -> Mux/2
  Mux/1 -> Product/2
  Sum/1 -> Trigonometric Function1/1
  Sum1/1 -> Product1/1
  Constant3/1 -> Product1/2
  Constant4/1 -> Sum1/2
  Product1/1 -> Sum6/2
  Constant/1 -> Sum/2
  Multiport Switch/1 -> Sum7/2
  Multiport Switch1/1 -> Sum3/2
  Multiport Switch2/1 -> Sum10/2
  Product/1 -> Demux/1
  Demux/1 -> 0<m<1 4/1  "T1"
  Demux/2 -> 0<m<1 5/1  "T2"
  Constant5/1 -> Sum4/1
  Sum4/1 -> 0<m<1 3/1  "T0"
  Gain1/1 -> Sum5/2
  Gain/1 -> Sum5/1, Multiport Switch/2, Multiport Switch/7, Multiport Switch1/3, Multiport Switch1/4, Multiport Switch2/5, Multiport Switch2/6  "cmp1"
  Sum5/1 -> Sum8/1, Multiport Switch1/5, Multiport Switch2/4, Multiport Switch2/7, Multiport Switch1/2, Multiport Switch/3, Multiport Switch/6  "cmp2"
  Gain2/1 -> Sum8/2
  Sum8/1 -> Multiport Switch/4, Multiport Switch/5, Multiport Switch1/6, Multiport Switch1/7, Multiport Switch2/2, Multiport Switch2/3  "cmp3"
  0<m<1 1/1 -> Gain2/1
  0<m<1 2/1 -> Gain1/1
  0<m<1 3/1 -> Gain/1
  Ubeta/1 -> Gain4/1
  Ualfa/1 -> Cartesian to Polar/2
  Gain3/1 -> Product/1
  Gain4/1 -> Cartesian to Polar/1
  Constant1/1 -> Math Function1/2
  Math Function1/1 -> Switch1/2
  Constant6/1 -> Sum9/2
  Sum9/1 -> Switch1/3
  Switch1/1 -> Trigonometric Function/1, Sum/1
  Sum6/1 -> Switch1/1, Sum9/1  "alpha1"
  0<m<1 4/1 -> Sum4/2, 0<m<1 2/1
  0<m<1 5/1 -> Sum4/3, 0<m<1 1/1

== system AM_07_model_pretvornik_FOC/Vzorcenje ==
  Constant : Constant  Value=Tstikalna/2
  Repeating Sequence : simulink/Sources/Repeating Sequence  rep_seq_t=[0 Tstikalna]  rep_seq_y=[0 Tstikalna]
  Sum : Sum  Inputs=+-
  trigger : Outport
  wires:
  Repeating Sequence/1 -> Sum/1
  Constant/1 -> Sum/2
  Sum/1 -> trigger/1

== system AM_07_model_pretvornik_FOC/ACIM_model/Elektricni del1 ==
  U_123 : Inport
  w_meh : Inport  Port=2
  Clarke : Subsystem
  Inverzni Clarke : Subsystem
  Inverzni Park : Subsystem
  Park : Subsystem
  napetostni dq model : Subsystem
  Mel : Outport
  I_123 : Outport  Port=2
  wires:
  Park/1(U_dq) -> napetostni dq model/1(Us_dq)
  Clarke/1(U_ab) -> Park/1(U_ab)
  napetostni dq model/3(ro) -> Park/2(kot), Inverzni Park/2(kot)
  napetostni dq model/2(Is_dq) -> Inverzni Park/1(I_dq)
  Inverzni Park/1(I_ab) -> Inverzni Clarke/1(I_ab)
  U_123/1 -> Clarke/1(U_123)
  Inverzni Clarke/1(I_123) -> I_123/1
  napetostni dq model/1(Mel) -> Mel/1
  w_meh/1 -> napetostni dq model/2(wr)

== system AM_07_model_pretvornik_FOC/ACIM_model/Mehanika ==
  M_el : Inport
  M_br : Inport  Port=2
  Integrator : Integrator
  Sum : Sum  Inputs=+--
  eq 2.19 : Subsystem
  trenje in zracni upor : Subsystem
  w_meh : Outport
  kot_meh : Outport  Port=2
  wires:
  eq 2.19/1(wr) -> w_meh/1, trenje in zracni upor/1(wr), Integrator/1
  M_el/1 -> Sum/1
  Sum/1 -> eq 2.19/1(M)
  M_br/1 -> Sum/2
  trenje in zracni upor/1(Mtrenja) -> Sum/3
  Integrator/1 -> kot_meh/1

== system AM_07_model_pretvornik_FOC/ACIM_model1/Elektricni del1 ==
  U_123 : Inport
  w_meh : Inport  Port=2
  Clarke : Subsystem
  Inverzni Clarke : Subsystem
  Inverzni Park : Subsystem
  Park : Subsystem
  napetostni dq model : Subsystem
  Mel : Outport
  I_123 : Outport  Port=2
  wires:
  w_meh/1 -> napetostni dq model/2(wr)
  napetostni dq model/1(Mel) -> Mel/1
  Inverzni Clarke/1(I_123) -> I_123/1
  U_123/1 -> Clarke/1(U_123)
  Inverzni Park/1(I_ab) -> Inverzni Clarke/1(I_ab)
  napetostni dq model/2(Is_dq) -> Inverzni Park/1(I_dq)
  napetostni dq model/3(ro) -> Inverzni Park/2(kot), Park/2(kot)
  Clarke/1(U_ab) -> Park/1(U_ab)
  Park/1(U_dq) -> napetostni dq model/1(Us_dq)

== system AM_07_model_pretvornik_FOC/ACIM_model1/Mehanika ==
  M_el : Inport
  M_br : Inport  Port=2
  Integrator : Integrator
  Sum : Sum  Inputs=+--
  eq 2.19 : Subsystem
  trenje in zracni upor : Subsystem
  w_meh : Outport
  kot_meh : Outport  Port=2
  wires:
  Integrator/1 -> kot_meh/1
  trenje in zracni upor/1(Mtrenja) -> Sum/3
  M_br/1 -> Sum/2
  Sum/1 -> eq 2.19/1(M)
  M_el/1 -> Sum/1
  eq 2.19/1(wr) -> Integrator/1, trenje in zracni upor/1(wr), w_meh/1

== system AM_07_model_pretvornik_FOC/ACIM_model2/Elektricni del1 ==
  U_123 : Inport
  w_meh : Inport  Port=2
  Clarke : Subsystem
  Inverzni Clarke : Subsystem
  Inverzni Park : Subsystem
  Park : Subsystem
  napetostni dq model : Subsystem
  Mel : Outport
  I_123 : Outport  Port=2
  wires:
  Park/1(U_dq) -> napetostni dq model/1(Us_dq)
  Clarke/1(U_ab) -> Park/1(U_ab)
  napetostni dq model/3(ro) -> Park/2(kot), Inverzni Park/2(kot)
  napetostni dq model/2(Is_dq) -> Inverzni Park/1(I_dq)
  Inverzni Park/1(I_ab) -> Inverzni Clarke/1(I_ab)
  U_123/1 -> Clarke/1(U_123)
  Inverzni Clarke/1(I_123) -> I_123/1
  napetostni dq model/1(Mel) -> Mel/1
  w_meh/1 -> napetostni dq model/2(wr)

== system AM_07_model_pretvornik_FOC/ACIM_model2/Mehanika ==
  M_el : Inport
  M_br : Inport  Port=2
  Integrator : Integrator
  Sum : Sum  Inputs=+--
  eq 2.19 : Subsystem
  trenje in zracni upor : Subsystem
  w_meh : Outport
  kot_meh : Outport  Port=2
  wires:
  eq 2.19/1(wr) -> w_meh/1, trenje in zracni upor/1(wr), Integrator/1
  M_el/1 -> Sum/1
  Sum/1 -> eq 2.19/1(M)
  M_br/1 -> Sum/2
  trenje in zracni upor/1(Mtrenja) -> Sum/3
  Integrator/1 -> kot_meh/1

== system AM_07_model_pretvornik_FOC/Regulacija/Inverzni Park ==
  U_dq : Inport
  kot : Inport  Port=2
  Demux : Demux  Outputs=2
  Mux : Mux  Inputs=2
  "Sum1 " : Sum  Inputs=+-  SaturateOnIntegerOverflow=on  InputSameDT=on  OutDataTypeStr=Inherit: Same as first input
  Sum2 : Sum  SaturateOnIntegerOverflow=on  InputSameDT=on  OutDataTypeStr=Inherit: Same as first input
  cos : Fcn  Expr=cos(u)
  sin : Fcn  Expr=sin(u)
  x_d*cos : Product  SaturateOnIntegerOverflow=on  RndMeth=Zero  InputSameDT=on  OutDataTypeStr=Inherit: Same as first input
  x_d*sin : Product  SaturateOnIntegerOverflow=on  RndMeth=Zero  InputSameDT=on  OutDataTypeStr=Inherit: Same as first input
  x_q*cos : Product  SaturateOnIntegerOverflow=on  RndMeth=Zero  InputSameDT=on  OutDataTypeStr=Inherit: Same as first input
  "x_q*sin " : Product  SaturateOnIntegerOverflow=on  RndMeth=Zero  InputSameDT=on  OutDataTypeStr=Inherit: Same as first input
  U_ab : Outport
  wires:
  kot/1 -> sin/1, cos/1
  Sum2/1 -> Mux/2
  "Sum1 "/1 -> Mux/1
  x_d*sin/1 -> Sum2/1
  x_q*cos/1 -> Sum2/2
  "x_q*sin "/1 -> "Sum1 "/2
  x_d*cos/1 -> "Sum1 "/1
  sin/1 -> x_d*sin/2, "x_q*sin "/2
  cos/1 -> x_d*cos/2, x_q*cos/2
  Demux/2 -> x_q*cos/1, "x_q*sin "/1
  Demux/1 -> x_d*cos/1, x_d*sin/1
  U_dq/1 -> Demux/1
  Mux/1 -> U_ab/1

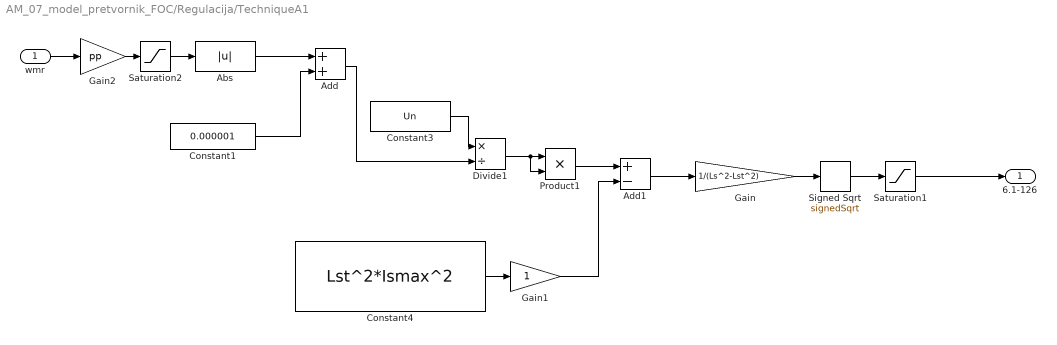
== system AM_07_model_pretvornik_FOC/Regulacija/TechniqueA1 ==
  wmr : Inport
  Abs : Abs
  Add : Sum
  Add1 : Sum  Inputs=+-
  Constant1 : Constant  Value=0.000001
  Constant3 : Constant  Value=Un
  Constant4 : Constant  Value=Lst^2*Ismax^2
  Divide1 : Product  Inputs=*/
  Gain : Gain  Gain=1/(Ls^2-Lst^2)
  Gain1 : Gain
  Gain2 : Gain  Gain=pp
  Product1 : Product
  Saturation1 : Saturate  UpperLimit=+Imrn*sqrt(2)  LowerLimit=-Imrn*sqrt(2)
  Saturation2 : Saturate  UpperLimit=wb_upper_limit_field_weaking  LowerLimit=-wb_upper_limit_field_weaking
  Signed Sqrt : Sqrt  Operator=signedSqrt  SaturateOnIntegerOverflow=on
  6.1-126 : Outport
  wires:
  Add/1 -> Divide1/2
  Abs/1 -> Add/1
  Constant1/1 -> Add/2
  Constant3/1 -> Divide1/1
  Divide1/1 -> Product1/2, Product1/1
  Product1/1 -> Add1/1
  Saturation1/1 -> 6.1-126/1
  Add1/1 -> Gain/1
  Gain/1 -> Signed Sqrt/1
  Signed Sqrt/1 -> Saturation1/1
  Saturation2/1 -> Abs/1
  Constant4/1 -> Gain1/1
  Gain1/1 -> Add1/2
  wmr/1 -> Gain2/1
  Gain2/1 -> Saturation2/1

== system AM_07_model_pretvornik_FOC/Regulacija/hitrostna regulacija ==
  ref : Inport
  fdb : Inport  Port=2
  1/Ti : Gain  Gain=Ki_wr  SaturateOnIntegerOverflow=on  OutDataTypeStr=Inherit: Same as input  ParamDataTypeStr=Inherit: Same as input
  Abs : Abs
  Add2 : Sum  Inputs=+-
  Compare To Zero : simulink/Logic and Bit Operations/Compare To Zero  relop=<=  OutDataTypeStr=boolean
  Discrete-Time Integrator : DiscreteIntegrator  SampleTime=-1  ICPrevOutput=DiscIntNeverNeededParam  ICPrevScaledInput=DiscIntNeverNeededParam
  Kp : Gain  Gain=Kp_wr  SaturateOnIntegerOverflow=on  OutDataTypeStr=Inherit: Same as input  ParamDataTypeStr=Inherit: Same as input
  Product : Product
  Saturation : Saturate  UpperLimit=+sqrt((In^2 - Imrn^2))*sqrt(2)  LowerLimit=-sqrt((In^2 - Imrn^2))*sqrt(2)
  Sum1 : Sum  Inputs=|+-
  Sum2 : Sum  Inputs=|++
  U_out : Outport
  wires:
  Saturation/1 -> Add2/2, U_out/1
  Kp/1 -> Sum2/1
  1/Ti/1 -> Discrete-Time Integrator/1
  Sum1/1 -> Product/1, Kp/1
  ref/1 -> Sum1/1
  fdb/1 -> Sum1/2
  Discrete-Time Integrator/1 -> Sum2/2
  Sum2/1 -> Add2/1, Saturation/1
  Add2/1 -> Abs/1
  Abs/1 -> Compare To Zero/1
  Compare To Zero/1 -> Product/2
  Product/1 -> 1/Ti/1

== system AM_07_model_pretvornik_FOC/Regulacija/tokovna regulacija d ==
  ref : Inport
  fdb : Inport  Port=2
  1/Ti : Gain  Gain=Ki_tok  SaturateOnIntegerOverflow=on  OutDataTypeStr=Inherit: Same as input  ParamDataTypeStr=Inherit: Same as input
  Abs : Abs
  Add2 : Sum  Inputs=+-
  Compare To Zero : simulink/Logic and Bit Operations/Compare To Zero  relop=<=  OutDataTypeStr=boolean
  Discrete-Time Integrator : DiscreteIntegrator  SampleTime=-1  ICPrevOutput=DiscIntNeverNeededParam  ICPrevScaledInput=DiscIntNeverNeededParam
  Kp : Gain  Gain=Kp_tok  SaturateOnIntegerOverflow=on  OutDataTypeStr=Inherit: Same as input  ParamDataTypeStr=Inherit: Same as input
  Product : Product
  Saturation : Saturate  UpperLimit=+0.99  LowerLimit=-0.99
  Sum1 : Sum  Inputs=|+-
  Sum2 : Sum  Inputs=|++
  out : Outport
  wires:
  Saturation/1 -> Add2/2, out/1
  Kp/1 -> Sum2/1
  1/Ti/1 -> Discrete-Time Integrator/1
  Sum1/1 -> Product/1, Kp/1
  ref/1 -> Sum1/1
  fdb/1 -> Sum1/2
  Discrete-Time Integrator/1 -> Sum2/2
  Sum2/1 -> Add2/1, Saturation/1
  Add2/1 -> Abs/1
  Abs/1 -> Compare To Zero/1
  Compare To Zero/1 -> Product/2
  Product/1 -> 1/Ti/1

== system AM_07_model_pretvornik_FOC/Regulacija/tokovna regulacija q ==
  ref : Inport
  fdb : Inport  Port=2
  1/Ti : Gain  Gain=Ki_tok  SaturateOnIntegerOverflow=on  OutDataTypeStr=Inherit: Same as input  ParamDataTypeStr=Inherit: Same as input
  Abs : Abs
  Add2 : Sum  Inputs=+-
  Compare To Zero : simulink/Logic and Bit Operations/Compare To Zero  relop=<=  OutDataTypeStr=boolean
  Discrete-Time Integrator : DiscreteIntegrator  SampleTime=-1  ICPrevOutput=DiscIntNeverNeededParam  ICPrevScaledInput=DiscIntNeverNeededParam
  Kp : Gain  Gain=Kp_tok  SaturateOnIntegerOverflow=on  OutDataTypeStr=Inherit: Same as input  ParamDataTypeStr=Inherit: Same as input
  Product : Product
  Saturation : Saturate  UpperLimit=+0.99  LowerLimit=-0.99
  Sum1 : Sum  Inputs=|+-
  Sum2 : Sum  Inputs=|++
  out : Outport
  wires:
  Saturation/1 -> Add2/2, out/1
  Kp/1 -> Sum2/1
  1/Ti/1 -> Discrete-Time Integrator/1
  Sum1/1 -> Product/1, Kp/1
  ref/1 -> Sum1/1
  fdb/1 -> Sum1/2
  Discrete-Time Integrator/1 -> Sum2/2
  Sum2/1 -> Add2/1, Saturation/1
  Add2/1 -> Abs/1
  Abs/1 -> Compare To Zero/1
  Compare To Zero/1 -> Product/2
  Product/1 -> 1/Ti/1

== system AM_07_model_pretvornik_FOC/Regulacija/tokovni_model ==
  I_123 : Inport
  wr : Inport  Port=2
  Clarke : Subsystem
  Demux : Demux  Outputs=2
  Discrete-Time Integrator : DiscreteIntegrator  SampleTime=-1  ICPrevOutput=DiscIntNeverNeededParam  ICPrevScaledInput=DiscIntNeverNeededParam
  Gain : Gain  Gain=pp
  Park : Subsystem
  Terminator : Terminator
  eq 5.39 : Subsystem
  eq 5.40 : Subsystem
  I_dq : Outport
  Imr : Outport  Port=2
  ro : Outport  Port=3
  wires:
  Park/1(U_dq) -> I_dq/1, Demux/1
  Clarke/1(U_ab) -> Park/1(U_ab)
  I_123/1 -> Clarke/1(U_123)
  Demux/1 -> eq 5.39/1(Isd)
  eq 5.39/1(Imr) -> eq 5.40/1(Imr), Imr/1
  Demux/2 -> eq 5.40/2(Isq)
  Gain/1 -> eq 5.40/3(wr_el)
  eq 5.40/1(wmr) -> Discrete-Time Integrator/1
  Discrete-Time Integrator/1 -> ro/1, Park/2(kot)
  eq 5.39/2(dImr/dt) -> Terminator/1
  wr/1 -> Gain/1

== system AM_07_model_pretvornik_FOC/Regulacija1/Inverzni Park ==
  U_dq : Inport
  kot : Inport  Port=2
  Demux : Demux  Outputs=2
  Mux : Mux  Inputs=2
  "Sum1 " : Sum  Inputs=+-  SaturateOnIntegerOverflow=on  InputSameDT=on  OutDataTypeStr=Inherit: Same as first input
  Sum2 : Sum  SaturateOnIntegerOverflow=on  InputSameDT=on  OutDataTypeStr=Inherit: Same as first input
  cos : Fcn  Expr=cos(u)
  sin : Fcn  Expr=sin(u)
  x_d*cos : Product  SaturateOnIntegerOverflow=on  RndMeth=Zero  InputSameDT=on  OutDataTypeStr=Inherit: Same as first input
  x_d*sin : Product  SaturateOnIntegerOverflow=on  RndMeth=Zero  InputSameDT=on  OutDataTypeStr=Inherit: Same as first input
  x_q*cos : Product  SaturateOnIntegerOverflow=on  RndMeth=Zero  InputSameDT=on  OutDataTypeStr=Inherit: Same as first input
  "x_q*sin " : Product  SaturateOnIntegerOverflow=on  RndMeth=Zero  InputSameDT=on  OutDataTypeStr=Inherit: Same as first input
  U_ab : Outport
  wires:
  Mux/1 -> U_ab/1
  U_dq/1 -> Demux/1
  Demux/1 -> x_d*sin/1, x_d*cos/1
  Demux/2 -> "x_q*sin "/1, x_q*cos/1
  cos/1 -> x_q*cos/2, x_d*cos/2
  sin/1 -> "x_q*sin "/2, x_d*sin/2
  x_d*cos/1 -> "Sum1 "/1
  "x_q*sin "/1 -> "Sum1 "/2
  x_q*cos/1 -> Sum2/2
  x_d*sin/1 -> Sum2/1
  "Sum1 "/1 -> Mux/1
  Sum2/1 -> Mux/2
  kot/1 -> cos/1, sin/1

== system AM_07_model_pretvornik_FOC/Regulacija1/TechniqueB1 ==
  w : Inport
  Isdq : Inport  Port=2
  Imr : Inport  Port=3
  Add4 : Sum
  Const c : Subsystem
  Deljeno imenovalec 6.1-135 : Gain  Gain=1/(Ls^2-Lst^2)
  Demux : Demux  Outputs=2
  Gain4 : Gain  Gain=-Ls
  Gain6 : Gain  Gain=pp
  Korenski del : Subsystem
  Saturation : Saturate  UpperLimit=+Imrn*sqrt(2)  LowerLimit=-Imrn*sqrt(2)
  Terminator : Terminator
  6.1-135 : Outport
  wires:
  Demux/1 -> Const c/1(Id)
  Demux/2 -> Terminator/1
  Saturation/1 -> 6.1-135/1
  Const c/1(c) -> Korenski del/1(c), Gain4/1
  Gain4/1 -> Add4/1
  Add4/1 -> Deljeno imenovalec 6.1-135/1
  Deljeno imenovalec 6.1-135/1 -> Saturation/1
  Isdq/1 -> Demux/1
  Korenski del/1(korenjen del) -> Add4/2
  w/1 -> Gain6/1
  Gain6/1 -> Korenski del/2(w)
  Imr/1 -> Const c/2(Imr)

== system AM_07_model_pretvornik_FOC/Regulacija1/hitrostna regulacija ==
  ref : Inport
  fdb : Inport  Port=2
  1/Ti : Gain  Gain=Ki_wr  SaturateOnIntegerOverflow=on  OutDataTypeStr=Inherit: Same as input  ParamDataTypeStr=Inherit: Same as input
  Abs : Abs
  Add2 : Sum  Inputs=+-
  Compare To Zero : simulink/Logic and Bit Operations/Compare To Zero  relop=<=  OutDataTypeStr=boolean
  Discrete-Time Integrator : DiscreteIntegrator  SampleTime=-1  ICPrevOutput=DiscIntNeverNeededParam  ICPrevScaledInput=DiscIntNeverNeededParam
  Kp : Gain  Gain=Kp_wr  SaturateOnIntegerOverflow=on  OutDataTypeStr=Inherit: Same as input  ParamDataTypeStr=Inherit: Same as input
  Product : Product
  Saturation : Saturate  UpperLimit=+sqrt((In^2 - Imrn^2))*sqrt(2)  LowerLimit=-sqrt((In^2 - Imrn^2))*sqrt(2)
  Sum1 : Sum  Inputs=|+-
  Sum2 : Sum  Inputs=|++
  U_out : Outport
  wires:
  Product/1 -> 1/Ti/1
  Compare To Zero/1 -> Product/2
  Abs/1 -> Compare To Zero/1
  Add2/1 -> Abs/1
  Sum2/1 -> Saturation/1, Add2/1
  Discrete-Time Integrator/1 -> Sum2/2
  fdb/1 -> Sum1/2
  ref/1 -> Sum1/1
  Sum1/1 -> Kp/1, Product/1
  1/Ti/1 -> Discrete-Time Integrator/1
  Kp/1 -> Sum2/1
  Saturation/1 -> U_out/1, Add2/2

== system AM_07_model_pretvornik_FOC/Regulacija1/tokovna regulacija d ==
  ref : Inport
  fdb : Inport  Port=2
  1/Ti : Gain  Gain=Ki_tok  SaturateOnIntegerOverflow=on  OutDataTypeStr=Inherit: Same as input  ParamDataTypeStr=Inherit: Same as input
  Abs : Abs
  Add2 : Sum  Inputs=+-
  Compare To Zero : simulink/Logic and Bit Operations/Compare To Zero  relop=<=  OutDataTypeStr=boolean
  Discrete-Time Integrator : DiscreteIntegrator  SampleTime=-1  ICPrevOutput=DiscIntNeverNeededParam  ICPrevScaledInput=DiscIntNeverNeededParam
  Kp : Gain  Gain=Kp_tok  SaturateOnIntegerOverflow=on  OutDataTypeStr=Inherit: Same as input  ParamDataTypeStr=Inherit: Same as input
  Product : Product
  Saturation : Saturate  UpperLimit=+0.99  LowerLimit=-0.99
  Sum1 : Sum  Inputs=|+-
  Sum2 : Sum  Inputs=|++
  out : Outport
  wires:
  Product/1 -> 1/Ti/1
  Compare To Zero/1 -> Product/2
  Abs/1 -> Compare To Zero/1
  Add2/1 -> Abs/1
  Sum2/1 -> Saturation/1, Add2/1
  Discrete-Time Integrator/1 -> Sum2/2
  fdb/1 -> Sum1/2
  ref/1 -> Sum1/1
  Sum1/1 -> Kp/1, Product/1
  1/Ti/1 -> Discrete-Time Integrator/1
  Kp/1 -> Sum2/1
  Saturation/1 -> out/1, Add2/2

== system AM_07_model_pretvornik_FOC/Regulacija1/tokovna regulacija q ==
  ref : Inport
  fdb : Inport  Port=2
  1/Ti : Gain  Gain=Ki_tok  SaturateOnIntegerOverflow=on  OutDataTypeStr=Inherit: Same as input  ParamDataTypeStr=Inherit: Same as input
  Abs : Abs
  Add2 : Sum  Inputs=+-
  Compare To Zero : simulink/Logic and Bit Operations/Compare To Zero  relop=<=  OutDataTypeStr=boolean
  Discrete-Time Integrator : DiscreteIntegrator  SampleTime=-1  ICPrevOutput=DiscIntNeverNeededParam  ICPrevScaledInput=DiscIntNeverNeededParam
  Kp : Gain  Gain=Kp_tok  SaturateOnIntegerOverflow=on  OutDataTypeStr=Inherit: Same as input  ParamDataTypeStr=Inherit: Same as input
  Product : Product
  Saturation : Saturate  UpperLimit=+0.99  LowerLimit=-0.99
  Sum1 : Sum  Inputs=|+-
  Sum2 : Sum  Inputs=|++
  out : Outport
  wires:
  Product/1 -> 1/Ti/1
  Compare To Zero/1 -> Product/2
  Abs/1 -> Compare To Zero/1
  Add2/1 -> Abs/1
  Sum2/1 -> Saturation/1, Add2/1
  Discrete-Time Integrator/1 -> Sum2/2
  fdb/1 -> Sum1/2
  ref/1 -> Sum1/1
  Sum1/1 -> Kp/1, Product/1
  1/Ti/1 -> Discrete-Time Integrator/1
  Kp/1 -> Sum2/1
  Saturation/1 -> out/1, Add2/2
